simulink model "Modele_1"  (R2025b)
settings: Solver=VariableStepAuto  StartTime=0.0  StopTime=3  RelTol=1e-3
values from neighbouring files (symbols this model uses):
  d2 = 3.73    [variables.m]
  k = k + nzb    [kron.m]    (also in variables.m = 400)
  km = 2.96    [variables.m]
  ky = 280    [variables.m]
  m1 = 2.29    [variables.m]
  m2 = 2.044    [variables.m]
undefined symbols (not defined in the file or in its folder): d1
settings Model: Creator=Mohamed Yagoubi  LastModifiedBy=Mohamed Yagoubi

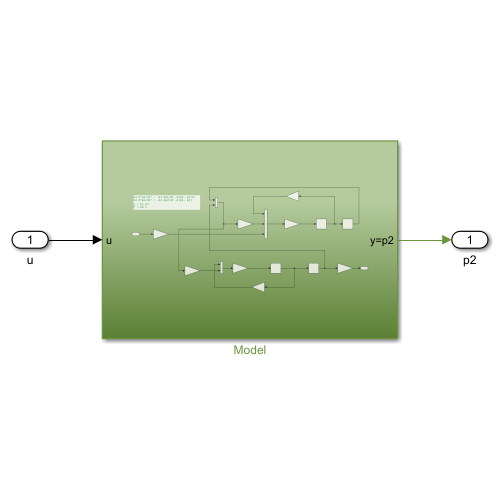
[thumbnail: Simulink's stored preview of the top-level diagram]
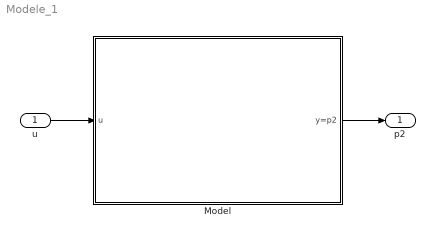
== system Modele_1 ==
  u : Inport
  Model : Subsystem
  p2 : Outport
  wires:
  u/1 -> Model/1(u)
  Model/1(y=p2) -> p2/1

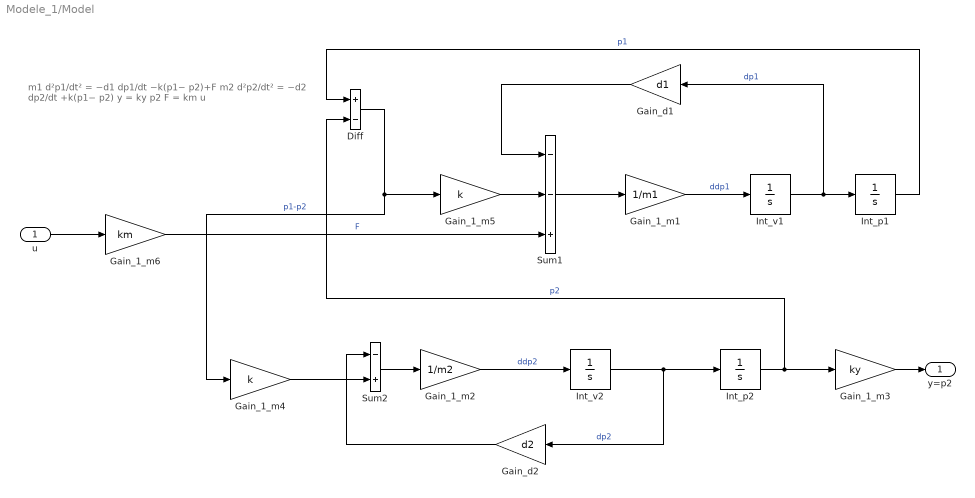
== system Modele_1/Model ==
  note: m1 d²p1/dt² = −d1 dp1/dt −k(p1− p2)+F
      | m2 d²p2/dt² = −d2 dp2/dt +k(p1− p2)
      | y = ky p2
      | F = km u
  u : Inport
  Diff : Sum  Inputs=+-
  Gain_1_m1 : Gain  Gain=1/m1
  Gain_1_m2 : Gain  Gain=1/m2
  Gain_1_m3 : Gain  Gain=ky
  Gain_1_m4 : Gain  Gain=k
  Gain_1_m5 : Gain  Gain=k
  Gain_1_m6 : Gain  Gain=km
  Gain_d1 : Gain  Gain=d1
  Gain_d2 : Gain  Gain=d2
  Int_p1 : Integrator
  Int_p2 : Integrator
  Int_v1 : Integrator
  Int_v2 : Integrator
  Sum1 : Sum  Inputs=--+
  Sum2 : Sum  Inputs=-+
  y=p2 : Outport
  wires:
  Int_v1/1 -> Gain_d1/1, Int_p1/1  "dp1"
  Diff/1 -> Gain_1_m4/1, Gain_1_m5/1  "p1-p2"
  Gain_d2/1 -> Sum2/1
  Gain_1_m1/1 -> Int_v1/1  "ddp1"
  Gain_d1/1 -> Sum1/1
  Int_v2/1 -> Gain_d2/1, Int_p2/1  "dp2"
  u/1 -> Gain_1_m6/1
  Sum2/1 -> Gain_1_m2/1
  Int_p2/1 -> Gain_1_m3/1, Diff/2  "p2"
  Gain_1_m2/1 -> Int_v2/1  "ddp2"
  Int_p1/1 -> Diff/1  "p1"
  Sum1/1 -> Gain_1_m1/1
  Gain_1_m3/1 -> y=p2/1
  Gain_1_m4/1 -> Sum2/2
  Gain_1_m5/1 -> Sum1/2
  Gain_1_m6/1 -> Sum1/3  "F"
